simulink model "untitled"  (R2016a)
settings: Solver=VariableStepAuto  StartTime=0.0  StopTime=100  RelTol=1e-3
values from neighbouring files (symbols this model uses):
  first_block = m*g*sin(Theta)    [calculatefx0.m]
  Fx0 = m*g*sin(Theta) + f*m*g + 0.5*rho*A*Cd*(u0+uw)^2    [calculatefx0.m]
  K = 68.5/m    (= 0.0685)    [calculatefx0.m]
  Ka = 10    [calculatefx0.m]
  m = 1000    [calculatefx0.m]
  second_block = f*m*g*cos(Theta)    [calculatefx0.m]
  Tau = 100    [calculatefx0.m]
  TauA = 0.05    [calculatefx0.m]
  third_block = 0.5*rho*A*Cd    (= 0.3005)    [calculatefx0.m]
  uc = 30    [calculatefx0.m]
  uw = 2    [calculatefx0.m]
settings Model: Creator=dumea  LastModifiedBy=dumea

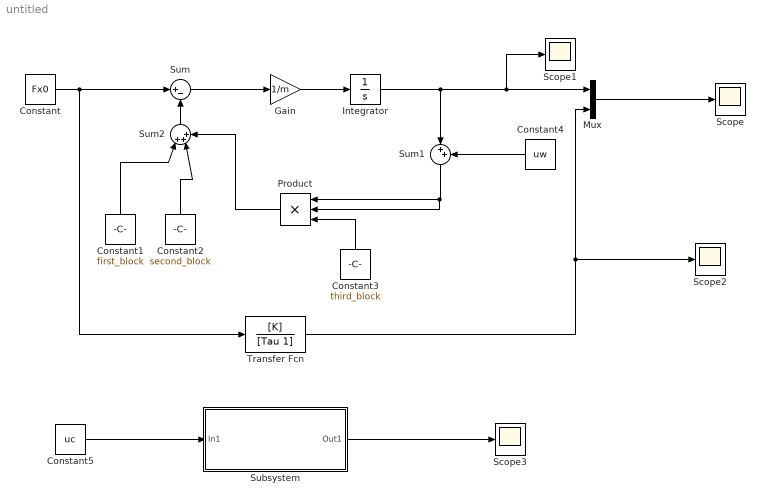
== system untitled ==
  Constant : Constant  Value=Fx0
  Constant1 : Constant  Value=first_block
  Constant2 : Constant  Value=second_block
  Constant3 : Constant  Value=third_block
  Constant4 : Constant  Value=uw
  Constant5 : Constant  Value=uc
  Gain : Gain  Gain=1/m
  Integrator : Integrator
  Mux : Mux  Inputs=2
  Product : Product  Inputs=3
  Scope{,1..3} (4 alike) : Scope
  Subsystem : Subsystem
  Sum : Sum  Inputs=|+-
  Sum1 : Sum  Inputs=|++
  Sum2 : Sum  Inputs=|+++
  Transfer Fcn : TransferFcn  Numerator=[K]  Denominator=[Tau 1]
  wires:
  Sum/1 -> Gain/1
  Gain/1 -> Integrator/1
  Integrator/1 -> Scope1/1, Mux/1, Sum1/1
  Constant3/1 -> Product/3
  Constant4/1 -> Sum1/2
  Sum1/1 -> Product/2, Product/1
  Product/1 -> Sum2/3
  Constant2/1 -> Sum2/2
  Constant1/1 -> Sum2/1
  Sum2/1 -> Sum/2
  Mux/1 -> Scope/1
  Constant/1 -> Transfer Fcn/1, Sum/1
  Transfer Fcn/1 -> Mux/2, Scope2/1
  Constant5/1 -> Subsystem/1(In1)
  Subsystem/1(Out1) -> Scope3/1

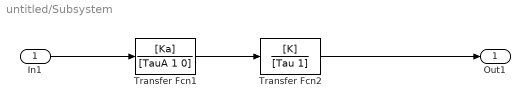
== system untitled/Subsystem ==
  In1 : Inport
  Transfer Fcn1 : TransferFcn  Numerator=[Ka]  Denominator=[TauA 1 0]
  Transfer Fcn2 : TransferFcn  Numerator=[K]  Denominator=[Tau 1]
  Out1 : Outport
  wires:
  Transfer Fcn2/1 -> Out1/1
  In1/1 -> Transfer Fcn1/1
  Transfer Fcn1/1 -> Transfer Fcn2/1
